simulink model "MLIB_ShBiSat_BAM_F16"  (Simulink 7.3)
settings: Solver=ode45  StartTime=0.0  StopTime=10.0  RelTol=1e-3
settings Model: Creator=B17364  LastModifiedBy=B17364

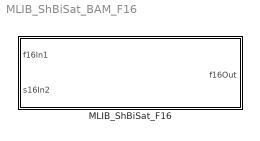
== system MLIB_ShBiSat_BAM_F16 ==
  MLIB_ShBiSat_F16 : Subsystem  mask(MLIB_ShBiSat_F16){}
      mask help: Bit accurate model of the fuction shifts the first parameter to left or right by number defined by second parameter and saturate if necessary. If the sign of second parameter is negative, shift to right. All parameters as well as input and output are 16bit integers.
      mask init:
      | pos = get_param(gcb, 'Position');width = pos(3) - pos(1); height = pos(4) - pos(2);tX=width/2;tY=height*0.9;
      mask Display: color('black');port_label('input',1,'f16In1');port_label('input',2,'s16In2');port_label('output',1,'f16Out');color('black');disp('MLIB_ShBiSat_F16');color('blue');text(tX,tY, 'BAM', 'horizontalAlignment', 'center');

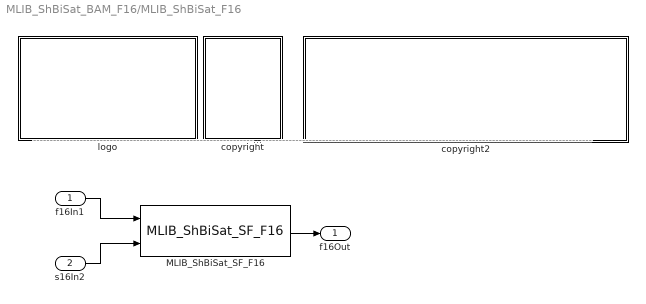
== system MLIB_ShBiSat_BAM_F16/MLIB_ShBiSat_F16 ==
  note: ---------------------------------------------------------------------------------------------------------------------------------------------------------------------------------------------------
  f16In1 : Inport  OutDataType=fixdt(1, 16)  OutScaling=2^0
  s16In2 : Inport  Port=2  OutDataType=fixdt(1, 16)  OutScaling=2^0
  MLIB_ShBiSat_SF_F16 : S-Function  FunctionName=MLIB_ShBiSat_SF_F16  EnableBusSupport=off
  copyright : Subsystem
      mask Display: text(10,90,'FILE:');text(10,75,'DESRIPTION:')text(10,60,'COPYRIGHT:')text(10,45,'VERSION:')text(10,30,'DATE:')
  copyright2 : Subsystem
      mask Display: text(10,90,'MLIB_ShBiSat_BAM_F16.mdl');text(10,75,'Shift the first parameter to left or right and saturate if necessary.');text(10,60,'Freescale')text(10,45,'0.1');text(10,30,'26-Aug-2011');
  logo : Subsystem
      mask Display: image(imread('logo.jpg'))
  f16Out : Outport  OutDataType=fixdt(1, 16)  OutScaling=2^0
  wires:
  f16In1/1 -> MLIB_ShBiSat_SF_F16/1
  s16In2/1 -> MLIB_ShBiSat_SF_F16/2
  MLIB_ShBiSat_SF_F16/1 -> f16Out/1

== system MLIB_ShBiSat_BAM_F16/MLIB_ShBiSat_F16/copyright ==

== system MLIB_ShBiSat_BAM_F16/MLIB_ShBiSat_F16/copyright2 ==

== system MLIB_ShBiSat_BAM_F16/MLIB_ShBiSat_F16/logo ==
